simulink model "labeca_simulink"  (R2023a)
settings: Solver=VariableStepAuto  StartTime=0.0  StopTime=0.6  RelTol=1e-3
values from neighbouring files (symbols this model uses):
  ganho_K = step_resposta/step_excitacao    [labeca.m]    (also in resposta_ao_degrau.m)
  tau_area = A0/(media_canal2_sup - media_canal2_inf)    [labeca.m]    (also in resposta_ao_degrau.m)
  tau_nep = 1 / a    [labeca.m]    (also in resposta_ao_degrau.m)
libraries: simulink x1
settings Model: Creator=helenabrener  LastModifiedBy=helenabrener

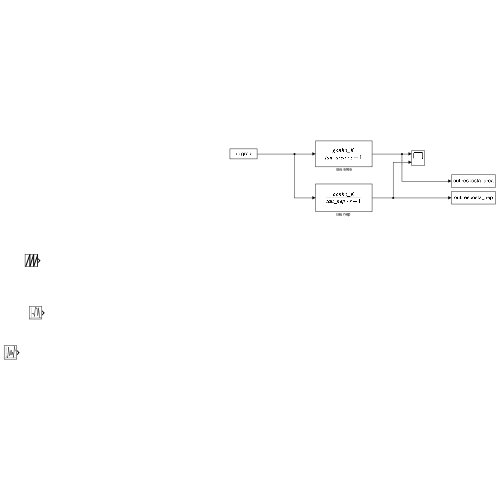
[thumbnail: Simulink's stored preview of the top-level diagram]
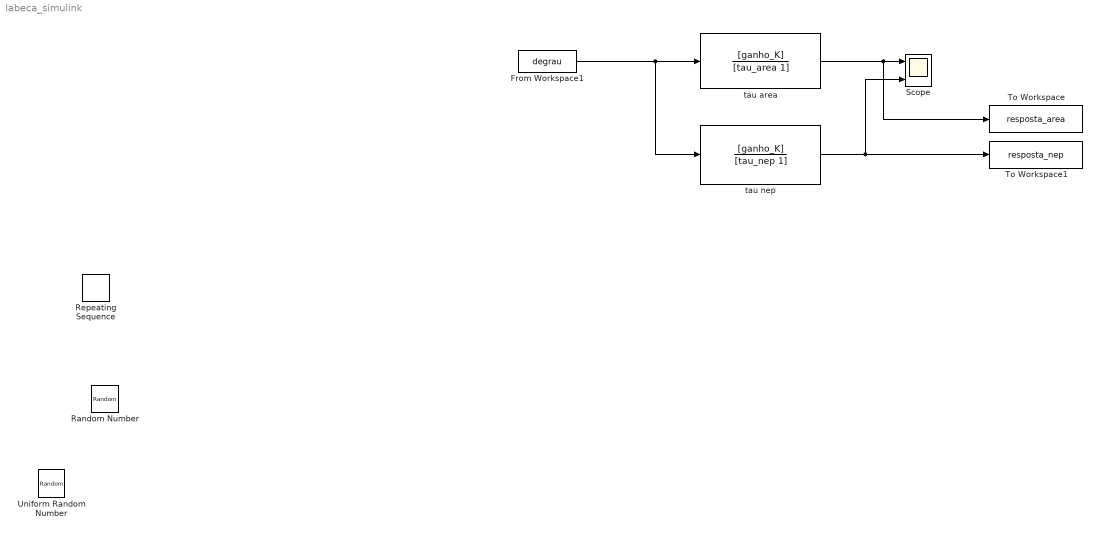
== system labeca_simulink ==
  " tau area" : TransferFcn  Numerator=[ganho_K]  Denominator=[tau_area 1]
  From Workspace1 : FromWorkspace  VariableName=degrau
  Random Number : RandomNumber  SampleTime=0.1
  Repeating Sequence : simulink/Sources/Repeating Sequence  rep_seq_t=[0 2]  rep_seq_y=[0 2]
  Scope : Scope  NumInputPorts=2
  To Workspace : ToWorkspace  VariableName=resposta_area  SaveFormat=Timeseries  SampleTime=-1
  To Workspace1 : ToWorkspace  VariableName=resposta_nep  SaveFormat=Timeseries  SampleTime=-1
  Uniform Random Number : UniformRandomNumber  SampleTime=0.1
  tau nep : TransferFcn  Numerator=[ganho_K]  Denominator=[tau_nep 1]
  wires:
  " tau area"/1 -> To Workspace/1, Scope/1
  tau nep/1 -> Scope/2, To Workspace1/1
  From Workspace1/1 -> tau nep/1, " tau area"/1
